simulink model "MultiIntersectionStoplight"  (R2020a)
settings: Solver=VariableStepAuto  StartTime=0.0  StopTime=inf  RelTol=1e-3
libraries: dspnetwork x119, sldrtlib x1
settings Model: Creator=brandon  LastModifiedBy=brandon

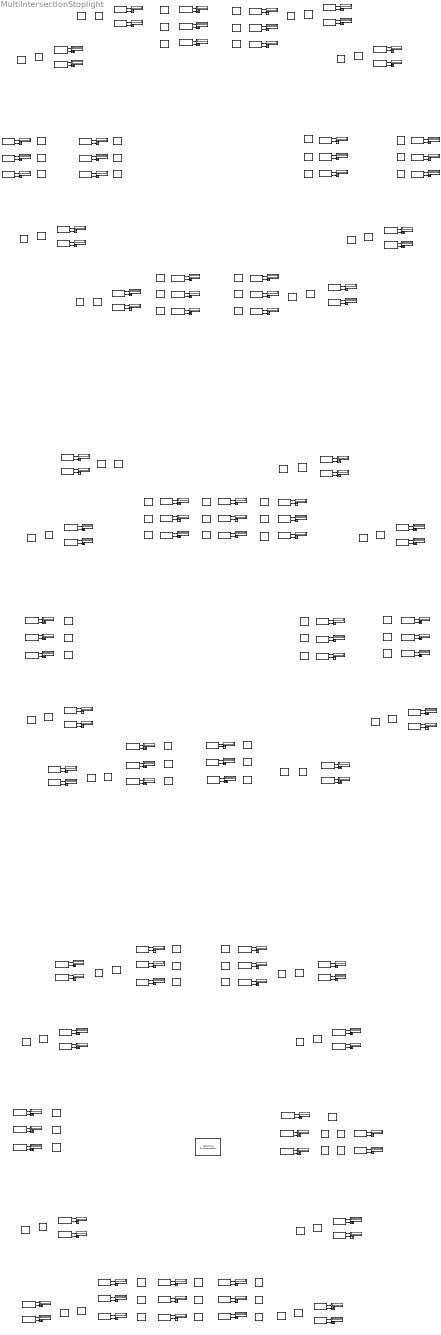
== system MultiIntersectionStoplight ==
  note: Walk: UDP 25003
      | Don't Walk: UDP 25004
  note: Walk: UDP 25005
      | Don't Walk: UDP 25006
  note: Walk: UDP 25011
      | Don't Walk: UDP 25012
  note: Walk: UDP 25013
      | Don't Walk: UDP 25014
  note: Red: UDP 26001
      | Yellow: UDP 26002
      | Green: UDP 26003
  note: Red: UDP 26004
      | Yellow: UDP 26005
      | Green: UDP 26006
  note: Red: UDP 26007
      | Yellow: UDP 26008
      | Green: UDP 26009
  note: Red: UDP 26010
      | Yellow: UDP 26011
      | Green: UDP 26012
  note: Red: UDP 26013
      | Yellow: UDP 26014
      | Green: UDP 26015
  note: Red: UDP 26016
      | Yellow: UDP 26017
      | Green: UDP 26018
  note: Red: UDP 26019
      | Yellow: UDP 26020
      | Green: UDP 26021
      | Yellow Left: UDP 26022
      | Green Left: UDP 26023
  note: Intersection of Ruggles and Huntington
      | Crosswalks: UDP Ports 25001-25016
      | Stoplights: UPD Ports 26001-26023
  note: Intersection of Parker and Huntington
      | Crosswalks: UDP Ports 25017-25032
      | Stoplights: UPD Ports 26024-26047
  note: Walk: UDP 25019
      | Don't Walk: UDP 25020
  note: Walk: UDP 25021
      | Don't Walk: UDP 25022
  note: Walk: UDP 25029
      | Don't Walk: UDP 25030
  note: Walk: UDP 25027
      | Don't Walk: UDP 25028
  note: Red: UDP 26024
      | Yellow: UDP 26025
      | Green: UDP 26026
  note: Red: UDP 26027
      | Yellow: UDP 26028
      | Green: UDP 26029
  note: Red: UDP 26030
      | Yellow: UDP 26031
      | Green: UDP 26032
  note: Red: UDP 26033
      | Yellow: UDP 26034
      | Green: UDP 26035
  note: Red: UDP 26036
      | Yellow: UDP 26037
      | Green: UDP 26038
  note: Red: UDP 26039
      | Yellow: UDP 26040
      | Green: UDP 26041
  note: Red: UDP 26042
      | Yellow: UDP 26043
      | Green: UDP 26044
  note: Red: UDP 26045
      | Yellow: UDP 26046
      | Green: UDP 26047
  note: Intersection of Parker and Huntington
      | Crosswalks: UDP Ports 25033-25048
      | Stoplights: UPD Ports 26048-26071
  note: Walk: UDP 25035
      | Don't Walk: UDP 25036
  note: Walk: UDP 25037
      | Don't Walk: UDP 25038
  note: Walk: UDP 25045
      | Don't Walk: UDP 25046
  note: Walk: UDP 25043
      | Don't Walk: UDP 25044
  note: Red: UDP 26066
      | Yellow: UDP 26067
      | Green: UDP 26068
  note: Red: UDP 26069
      | Yellow: UDP 26070
      | Green: UDP 26071
  note: Red: UDP 26048
      | Yellow: UDP 26049
      | Green: UDP 26050
  note: Red: UDP 26051
      | Yellow: UDP 26052
      | Green: UDP 26053
  note: Red: UDP 26057
      | Yellow: UDP 26058
      | Green: UDP 26059
  note: Red: UDP 26054
      | Yellow: UDP 26055
      | Green: UDP 26056
  note: Red: UDP 26060
      | Yellow: UDP 26061
      | Green: UDP 26062
  note: Red: UDP 26063
      | Yellow: UDP 26064
      | Green: UDP 26065
  note: Walk: UDP 25001
      | Don't Walk: UDP 25002
  note: Walk: UDP 25015
      | Don't Walk: UDP 25016
  note: Walk: UDP 25009
      | Don't Walk: UDP 25010
  note: Walk: UDP 25007
      | Don't Walk: UDP 25008
  note: Walk: UDP 25025
      | Don't Walk: UDP 25026
  note: Walk: UDP 25031
      | Don't Walk: UDP 25032
  note: Walk: UDP 25017
      | Don't Walk: UDP 25018
  note: Walk: UDP 25023
      | Don't Walk: UDP 25024
  note: Walk: UDP 25047
      | Don't Walk: UDP 25048
  note: Walk: UDP 25033
      | Don't Walk: UDP 25034
  note: Walk: UDP 25039
      | Don't Walk: UDP 25040
  note: Walk: UDP 25041
      | Don't Walk: UDP 25042
  Display{1..119} (119 alike) : Display
  Lamp{1..119} (119 alike) : LampBlock  LabelPosition=Hide
  Real-Time Synchronization : sldrtlib/Real-Time Synchronization  SampleTime=0.1  MaxMissedTicks=1000000  ShowMissedTicks=off  YieldWhenWaiting=off
  Terminator{1..119} (119 alike) : Terminator
  UDP Receive1 : dspnetwork/UDP Receive  localURL='0.0.0.0'  localPort=26010  remoteURL='0.0.0.0'  remotePort=-1  recvBufferSize=2  dims=1  signalDatatype=uint16  isComplex=off  isVarSize=off  showBlockingTime=off  blockingTime=0  sampletime=0.1  blockPlatform=[]
  UDP Receive10 : dspnetwork/UDP Receive  localURL='0.0.0.0'  localPort=26016  remoteURL='0.0.0.0'  remotePort=-1  recvBufferSize=2  dims=1  signalDatatype=uint16  isComplex=off  isVarSize=off  showBlockingTime=off  blockingTime=0  sampletime=0.1  blockPlatform=[]
  UDP Receive100 : dspnetwork/UDP Receive  localURL='0.0.0.0'  localPort=25009  remoteURL='0.0.0.0'  remotePort=-1  recvBufferSize=2  dims=1  signalDatatype=uint16  isComplex=off  isVarSize=off  showBlockingTime=off  blockingTime=0  sampletime=0.1  blockPlatform=[]
  UDP Receive101 : dspnetwork/UDP Receive  localURL='0.0.0.0'  localPort=25010  remoteURL='0.0.0.0'  remotePort=-1  recvBufferSize=2  dims=1  signalDatatype=uint16  isComplex=off  isVarSize=off  showBlockingTime=off  blockingTime=0  sampletime=0.1  blockPlatform=[]
  UDP Receive102 : dspnetwork/UDP Receive  localURL='0.0.0.0'  localPort=25007  remoteURL='0.0.0.0'  remotePort=-1  recvBufferSize=2  dims=1  signalDatatype=uint16  isComplex=off  isVarSize=off  showBlockingTime=off  blockingTime=0  sampletime=0.1  blockPlatform=[]
  UDP Receive103 : dspnetwork/UDP Receive  localURL='0.0.0.0'  localPort=25008  remoteURL='0.0.0.0'  remotePort=-1  recvBufferSize=2  dims=1  signalDatatype=uint16  isComplex=off  isVarSize=off  showBlockingTime=off  blockingTime=0  sampletime=0.1  blockPlatform=[]
  UDP Receive104 : dspnetwork/UDP Receive  localURL='0.0.0.0'  localPort=25025  remoteURL='0.0.0.0'  remotePort=-1  recvBufferSize=2  dims=1  signalDatatype=uint16  isComplex=off  isVarSize=off  showBlockingTime=off  blockingTime=0  sampletime=0.1  blockPlatform=[]
  UDP Receive105 : dspnetwork/UDP Receive  localURL='0.0.0.0'  localPort=25026  remoteURL='0.0.0.0'  remotePort=-1  recvBufferSize=2  dims=1  signalDatatype=uint16  isComplex=off  isVarSize=off  showBlockingTime=off  blockingTime=0  sampletime=0.1  blockPlatform=[]
  UDP Receive106 : dspnetwork/UDP Receive  localURL='0.0.0.0'  localPort=25031  remoteURL='0.0.0.0'  remotePort=-1  recvBufferSize=2  dims=1  signalDatatype=uint16  isComplex=off  isVarSize=off  showBlockingTime=off  blockingTime=0  sampletime=0.1  blockPlatform=[]
  UDP Receive107 : dspnetwork/UDP Receive  localURL='0.0.0.0'  localPort=25032  remoteURL='0.0.0.0'  remotePort=-1  recvBufferSize=2  dims=1  signalDatatype=uint16  isComplex=off  isVarSize=off  showBlockingTime=off  blockingTime=0  sampletime=0.1  blockPlatform=[]
  UDP Receive108 : dspnetwork/UDP Receive  localURL='0.0.0.0'  localPort=25017  remoteURL='0.0.0.0'  remotePort=-1  recvBufferSize=2  dims=1  signalDatatype=uint16  isComplex=off  isVarSize=off  showBlockingTime=off  blockingTime=0  sampletime=0.1  blockPlatform=[]
  UDP Receive109 : dspnetwork/UDP Receive  localURL='0.0.0.0'  localPort=25018  remoteURL='0.0.0.0'  remotePort=-1  recvBufferSize=2  dims=1  signalDatatype=uint16  isComplex=off  isVarSize=off  showBlockingTime=off  blockingTime=0  sampletime=0.1  blockPlatform=[]
  UDP Receive11 : dspnetwork/UDP Receive  localURL='0.0.0.0'  localPort=26013  remoteURL='0.0.0.0'  remotePort=-1  recvBufferSize=2  dims=1  signalDatatype=uint16  isComplex=off  isVarSize=off  showBlockingTime=off  blockingTime=0  sampletime=0.1  blockPlatform=[]
  UDP Receive110 : dspnetwork/UDP Receive  localURL='0.0.0.0'  localPort=25023  remoteURL='0.0.0.0'  remotePort=-1  recvBufferSize=2  dims=1  signalDatatype=uint16  isComplex=off  isVarSize=off  showBlockingTime=off  blockingTime=0  sampletime=0.1  blockPlatform=[]
  UDP Receive111 : dspnetwork/UDP Receive  localURL='0.0.0.0'  localPort=25024  remoteURL='0.0.0.0'  remotePort=-1  recvBufferSize=2  dims=1  signalDatatype=uint16  isComplex=off  isVarSize=off  showBlockingTime=off  blockingTime=0  sampletime=0.1  blockPlatform=[]
  UDP Receive112 : dspnetwork/UDP Receive  localURL='0.0.0.0'  localPort=25047  remoteURL='0.0.0.0'  remotePort=-1  recvBufferSize=2  dims=1  signalDatatype=uint16  isComplex=off  isVarSize=off  showBlockingTime=off  blockingTime=0  sampletime=0.1  blockPlatform=[]
  UDP Receive113 : dspnetwork/UDP Receive  localURL='0.0.0.0'  localPort=25048  remoteURL='0.0.0.0'  remotePort=-1  recvBufferSize=2  dims=1  signalDatatype=uint16  isComplex=off  isVarSize=off  showBlockingTime=off  blockingTime=0  sampletime=0.1  blockPlatform=[]
  UDP Receive114 : dspnetwork/UDP Receive  localURL='0.0.0.0'  localPort=25033  remoteURL='0.0.0.0'  remotePort=-1  recvBufferSize=2  dims=1  signalDatatype=uint16  isComplex=off  isVarSize=off  showBlockingTime=off  blockingTime=0  sampletime=0.1  blockPlatform=[]
  UDP Receive115 : dspnetwork/UDP Receive  localURL='0.0.0.0'  localPort=25034  remoteURL='0.0.0.0'  remotePort=-1  recvBufferSize=2  dims=1  signalDatatype=uint16  isComplex=off  isVarSize=off  showBlockingTime=off  blockingTime=0  sampletime=0.1  blockPlatform=[]
  UDP Receive116 : dspnetwork/UDP Receive  localURL='0.0.0.0'  localPort=25039  remoteURL='0.0.0.0'  remotePort=-1  recvBufferSize=2  dims=1  signalDatatype=uint16  isComplex=off  isVarSize=off  showBlockingTime=off  blockingTime=0  sampletime=0.1  blockPlatform=[]
  UDP Receive117 : dspnetwork/UDP Receive  localURL='0.0.0.0'  localPort=25040  remoteURL='0.0.0.0'  remotePort=-1  recvBufferSize=2  dims=1  signalDatatype=uint16  isComplex=off  isVarSize=off  showBlockingTime=off  blockingTime=0  sampletime=0.1  blockPlatform=[]
  UDP Receive118 : dspnetwork/UDP Receive  localURL='0.0.0.0'  localPort=25041  remoteURL='0.0.0.0'  remotePort=-1  recvBufferSize=2  dims=1  signalDatatype=uint16  isComplex=off  isVarSize=off  showBlockingTime=off  blockingTime=0  sampletime=0.1  blockPlatform=[]
  UDP Receive119 : dspnetwork/UDP Receive  localURL='0.0.0.0'  localPort=25042  remoteURL='0.0.0.0'  remotePort=-1  recvBufferSize=2  dims=1  signalDatatype=uint16  isComplex=off  isVarSize=off  showBlockingTime=off  blockingTime=0  sampletime=0.1  blockPlatform=[]
  UDP Receive12 : dspnetwork/UDP Receive  localURL='0.0.0.0'  localPort=26007  remoteURL='0.0.0.0'  remotePort=-1  recvBufferSize=2  dims=1  signalDatatype=uint16  isComplex=off  isVarSize=off  showBlockingTime=off  blockingTime=0  sampletime=0.1  blockPlatform=[]
  UDP Receive13 : dspnetwork/UDP Receive  localURL='0.0.0.0'  localPort=26008  remoteURL='0.0.0.0'  remotePort=-1  recvBufferSize=2  dims=1  signalDatatype=uint16  isComplex=off  isVarSize=off  showBlockingTime=off  blockingTime=0  sampletime=0.1  blockPlatform=[]
  UDP Receive14 : dspnetwork/UDP Receive  localURL='0.0.0.0'  localPort=26009  remoteURL='0.0.0.0'  remotePort=-1  recvBufferSize=2  dims=1  signalDatatype=uint16  isComplex=off  isVarSize=off  showBlockingTime=off  blockingTime=0  sampletime=0.1  blockPlatform=[]
  UDP Receive15 : dspnetwork/UDP Receive  localURL='0.0.0.0'  localPort=26004  remoteURL='0.0.0.0'  remotePort=-1  recvBufferSize=2  dims=1  signalDatatype=uint16  isComplex=off  isVarSize=off  showBlockingTime=off  blockingTime=0  sampletime=0.1  blockPlatform=[]
  UDP Receive16 : dspnetwork/UDP Receive  localURL='0.0.0.0'  localPort=26005  remoteURL='0.0.0.0'  remotePort=-1  recvBufferSize=2  dims=1  signalDatatype=uint16  isComplex=off  isVarSize=off  showBlockingTime=off  blockingTime=0  sampletime=0.1  blockPlatform=[]
  UDP Receive17 : dspnetwork/UDP Receive  localURL='0.0.0.0'  localPort=26006  remoteURL='0.0.0.0'  remotePort=-1  recvBufferSize=2  dims=1  signalDatatype=uint16  isComplex=off  isVarSize=off  showBlockingTime=off  blockingTime=0  sampletime=0.1  blockPlatform=[]
  UDP Receive18 : dspnetwork/UDP Receive  localURL='0.0.0.0'  localPort=26001  remoteURL='0.0.0.0'  remotePort=-1  recvBufferSize=2  dims=1  signalDatatype=uint16  isComplex=off  isVarSize=off  showBlockingTime=off  blockingTime=0  sampletime=0.1  blockPlatform=[]
  UDP Receive19 : dspnetwork/UDP Receive  localURL='0.0.0.0'  localPort=26002  remoteURL='0.0.0.0'  remotePort=-1  recvBufferSize=2  dims=1  signalDatatype=uint16  isComplex=off  isVarSize=off  showBlockingTime=off  blockingTime=0  sampletime=0.1  blockPlatform=[]
  UDP Receive2 : dspnetwork/UDP Receive  localURL='0.0.0.0'  localPort=26011  remoteURL='0.0.0.0'  remotePort=-1  recvBufferSize=2  dims=1  signalDatatype=uint16  isComplex=off  isVarSize=off  showBlockingTime=off  blockingTime=0  sampletime=0.1  blockPlatform=[]
  UDP Receive20 : dspnetwork/UDP Receive  localURL='0.0.0.0'  localPort=26003  remoteURL='0.0.0.0'  remotePort=-1  recvBufferSize=2  dims=1  signalDatatype=uint16  isComplex=off  isVarSize=off  showBlockingTime=off  blockingTime=0  sampletime=0.1  blockPlatform=[]
  UDP Receive21 : dspnetwork/UDP Receive  localURL='0.0.0.0'  localPort=25005  remoteURL='0.0.0.0'  remotePort=-1  recvBufferSize=2  dims=1  signalDatatype=uint16  isComplex=off  isVarSize=off  showBlockingTime=off  blockingTime=0  sampletime=0.1  blockPlatform=[]
  UDP Receive22 : dspnetwork/UDP Receive  localURL='0.0.0.0'  localPort=25006  remoteURL='0.0.0.0'  remotePort=-1  recvBufferSize=2  dims=1  signalDatatype=uint16  isComplex=off  isVarSize=off  showBlockingTime=off  blockingTime=0  sampletime=0.1  blockPlatform=[]
  UDP Receive23 : dspnetwork/UDP Receive  localURL='0.0.0.0'  localPort=25003  remoteURL='0.0.0.0'  remotePort=-1  recvBufferSize=2  dims=1  signalDatatype=uint16  isComplex=off  isVarSize=off  showBlockingTime=off  blockingTime=0  sampletime=0.1  blockPlatform=[]
  UDP Receive24 : dspnetwork/UDP Receive  localURL='0.0.0.0'  localPort=25004  remoteURL='0.0.0.0'  remotePort=-1  recvBufferSize=2  dims=1  signalDatatype=uint16  isComplex=off  isVarSize=off  showBlockingTime=off  blockingTime=0  sampletime=0.1  blockPlatform=[]
  UDP Receive25 : dspnetwork/UDP Receive  localURL='0.0.0.0'  localPort=26021  remoteURL='0.0.0.0'  remotePort=-1  recvBufferSize=2  dims=1  signalDatatype=uint16  isComplex=off  isVarSize=off  showBlockingTime=off  blockingTime=0  sampletime=0.1  blockPlatform=[]
  UDP Receive26 : dspnetwork/UDP Receive  localURL='0.0.0.0'  localPort=26020  remoteURL='0.0.0.0'  remotePort=-1  recvBufferSize=2  dims=1  signalDatatype=uint16  isComplex=off  isVarSize=off  showBlockingTime=off  blockingTime=0  sampletime=0.1  blockPlatform=[]
  UDP Receive27 : dspnetwork/UDP Receive  localURL='0.0.0.0'  localPort=26023  remoteURL='0.0.0.0'  remotePort=-1  recvBufferSize=2  dims=1  signalDatatype=uint16  isComplex=off  isVarSize=off  showBlockingTime=off  blockingTime=0  sampletime=0.1  blockPlatform=[]
  UDP Receive28 : dspnetwork/UDP Receive  localURL='0.0.0.0'  localPort=26022  remoteURL='0.0.0.0'  remotePort=-1  recvBufferSize=2  dims=1  signalDatatype=uint16  isComplex=off  isVarSize=off  showBlockingTime=off  blockingTime=0  sampletime=0.1  blockPlatform=[]
  UDP Receive29 : dspnetwork/UDP Receive  localURL='0.0.0.0'  localPort=26019  remoteURL='0.0.0.0'  remotePort=-1  recvBufferSize=2  dims=1  signalDatatype=uint16  isComplex=off  isVarSize=off  showBlockingTime=off  blockingTime=0  sampletime=0.1  blockPlatform=[]
  UDP Receive3 : dspnetwork/UDP Receive  localURL='0.0.0.0'  localPort=25013  remoteURL='0.0.0.0'  remotePort=-1  recvBufferSize=2  dims=1  signalDatatype=uint16  isComplex=off  isVarSize=off  showBlockingTime=off  blockingTime=0  sampletime=0.1  blockPlatform=[]
  UDP Receive30 : dspnetwork/UDP Receive  localURL='0.0.0.0'  localPort=26014  remoteURL='0.0.0.0'  remotePort=-1  recvBufferSize=2  dims=1  signalDatatype=uint16  isComplex=off  isVarSize=off  showBlockingTime=off  blockingTime=0  sampletime=0.1  blockPlatform=[]
  UDP Receive31 : dspnetwork/UDP Receive  localURL='0.0.0.0'  localPort=26015  remoteURL='0.0.0.0'  remotePort=-1  recvBufferSize=2  dims=1  signalDatatype=uint16  isComplex=off  isVarSize=off  showBlockingTime=off  blockingTime=0  sampletime=0.1  blockPlatform=[]
  UDP Receive32 : dspnetwork/UDP Receive  localURL='0.0.0.0'  localPort=25019  remoteURL='0.0.0.0'  remotePort=-1  recvBufferSize=2  dims=1  signalDatatype=uint16  isComplex=off  isVarSize=off  showBlockingTime=off  blockingTime=0  sampletime=0.1  blockPlatform=[]
  UDP Receive33 : dspnetwork/UDP Receive  localURL='0.0.0.0'  localPort=25020  remoteURL='0.0.0.0'  remotePort=-1  recvBufferSize=2  dims=1  signalDatatype=uint16  isComplex=off  isVarSize=off  showBlockingTime=off  blockingTime=0  sampletime=0.1  blockPlatform=[]
  UDP Receive34 : dspnetwork/UDP Receive  localURL='0.0.0.0'  localPort=25021  remoteURL='0.0.0.0'  remotePort=-1  recvBufferSize=2  dims=1  signalDatatype=uint16  isComplex=off  isVarSize=off  showBlockingTime=off  blockingTime=0  sampletime=0.1  blockPlatform=[]
  UDP Receive35 : dspnetwork/UDP Receive  localURL='0.0.0.0'  localPort=25022  remoteURL='0.0.0.0'  remotePort=-1  recvBufferSize=2  dims=1  signalDatatype=uint16  isComplex=off  isVarSize=off  showBlockingTime=off  blockingTime=0  sampletime=0.1  blockPlatform=[]
  UDP Receive36 : dspnetwork/UDP Receive  localURL='0.0.0.0'  localPort=25027  remoteURL='0.0.0.0'  remotePort=-1  recvBufferSize=2  dims=1  signalDatatype=uint16  isComplex=off  isVarSize=off  showBlockingTime=off  blockingTime=0  sampletime=0.1  blockPlatform=[]
  UDP Receive37 : dspnetwork/UDP Receive  localURL='0.0.0.0'  localPort=25028  remoteURL='0.0.0.0'  remotePort=-1  recvBufferSize=2  dims=1  signalDatatype=uint16  isComplex=off  isVarSize=off  showBlockingTime=off  blockingTime=0  sampletime=0.1  blockPlatform=[]
  UDP Receive38 : dspnetwork/UDP Receive  localURL='0.0.0.0'  localPort=25029  remoteURL='0.0.0.0'  remotePort=-1  recvBufferSize=2  dims=1  signalDatatype=uint16  isComplex=off  isVarSize=off  showBlockingTime=off  blockingTime=0  sampletime=0.1  blockPlatform=[]
  UDP Receive39 : dspnetwork/UDP Receive  localURL='0.0.0.0'  localPort=25030  remoteURL='0.0.0.0'  remotePort=-1  recvBufferSize=2  dims=1  signalDatatype=uint16  isComplex=off  isVarSize=off  showBlockingTime=off  blockingTime=0  sampletime=0.1  blockPlatform=[]
  UDP Receive4 : dspnetwork/UDP Receive  localURL='0.0.0.0'  localPort=25014  remoteURL='0.0.0.0'  remotePort=-1  recvBufferSize=2  dims=1  signalDatatype=uint16  isComplex=off  isVarSize=off  showBlockingTime=off  blockingTime=0  sampletime=0.1  blockPlatform=[]
  UDP Receive40 : dspnetwork/UDP Receive  localURL='0.0.0.0'  localPort=26027  remoteURL='0.0.0.0'  remotePort=-1  recvBufferSize=2  dims=1  signalDatatype=uint16  isComplex=off  isVarSize=off  showBlockingTime=off  blockingTime=0  sampletime=0.1  blockPlatform=[]
  UDP Receive41 : dspnetwork/UDP Receive  localURL='0.0.0.0'  localPort=26028  remoteURL='0.0.0.0'  remotePort=-1  recvBufferSize=2  dims=1  signalDatatype=uint16  isComplex=off  isVarSize=off  showBlockingTime=off  blockingTime=0  sampletime=0.1  blockPlatform=[]
  UDP Receive42 : dspnetwork/UDP Receive  localURL='0.0.0.0'  localPort=26029  remoteURL='0.0.0.0'  remotePort=-1  recvBufferSize=2  dims=1  signalDatatype=uint16  isComplex=off  isVarSize=off  showBlockingTime=off  blockingTime=0  sampletime=0.1  blockPlatform=[]
  UDP Receive43 : dspnetwork/UDP Receive  localURL='0.0.0.0'  localPort=26024  remoteURL='0.0.0.0'  remotePort=-1  recvBufferSize=2  dims=1  signalDatatype=uint16  isComplex=off  isVarSize=off  showBlockingTime=off  blockingTime=0  sampletime=0.1  blockPlatform=[]
  UDP Receive44 : dspnetwork/UDP Receive  localURL='0.0.0.0'  localPort=26025  remoteURL='0.0.0.0'  remotePort=-1  recvBufferSize=2  dims=1  signalDatatype=uint16  isComplex=off  isVarSize=off  showBlockingTime=off  blockingTime=0  sampletime=0.1  blockPlatform=[]
  UDP Receive45 : dspnetwork/UDP Receive  localURL='0.0.0.0'  localPort=26026  remoteURL='0.0.0.0'  remotePort=-1  recvBufferSize=2  dims=1  signalDatatype=uint16  isComplex=off  isVarSize=off  showBlockingTime=off  blockingTime=0  sampletime=0.1  blockPlatform=[]
  UDP Receive46 : dspnetwork/UDP Receive  localURL='0.0.0.0'  localPort=26030  remoteURL='0.0.0.0'  remotePort=-1  recvBufferSize=2  dims=1  signalDatatype=uint16  isComplex=off  isVarSize=off  showBlockingTime=off  blockingTime=0  sampletime=0.1  blockPlatform=[]
  UDP Receive47 : dspnetwork/UDP Receive  localURL='0.0.0.0'  localPort=26031  remoteURL='0.0.0.0'  remotePort=-1  recvBufferSize=2  dims=1  signalDatatype=uint16  isComplex=off  isVarSize=off  showBlockingTime=off  blockingTime=0  sampletime=0.1  blockPlatform=[]
  UDP Receive48 : dspnetwork/UDP Receive  localURL='0.0.0.0'  localPort=26032  remoteURL='0.0.0.0'  remotePort=-1  recvBufferSize=2  dims=1  signalDatatype=uint16  isComplex=off  isVarSize=off  showBlockingTime=off  blockingTime=0  sampletime=0.1  blockPlatform=[]
  UDP Receive49 : dspnetwork/UDP Receive  localURL='0.0.0.0'  localPort=26044  remoteURL='0.0.0.0'  remotePort=-1  recvBufferSize=2  dims=1  signalDatatype=uint16  isComplex=off  isVarSize=off  showBlockingTime=off  blockingTime=0  sampletime=0.1  blockPlatform=[]
  UDP Receive5 : dspnetwork/UDP Receive  localURL='0.0.0.0'  localPort=26018  remoteURL='0.0.0.0'  remotePort=-1  recvBufferSize=2  dims=1  signalDatatype=uint16  isComplex=off  isVarSize=off  showBlockingTime=off  blockingTime=0  sampletime=0.1  blockPlatform=[]
  UDP Receive50 : dspnetwork/UDP Receive  localURL='0.0.0.0'  localPort=26043  remoteURL='0.0.0.0'  remotePort=-1  recvBufferSize=2  dims=1  signalDatatype=uint16  isComplex=off  isVarSize=off  showBlockingTime=off  blockingTime=0  sampletime=0.1  blockPlatform=[]
  UDP Receive51 : dspnetwork/UDP Receive  localURL='0.0.0.0'  localPort=26042  remoteURL='0.0.0.0'  remotePort=-1  recvBufferSize=2  dims=1  signalDatatype=uint16  isComplex=off  isVarSize=off  showBlockingTime=off  blockingTime=0  sampletime=0.1  blockPlatform=[]
  UDP Receive52 : dspnetwork/UDP Receive  localURL='0.0.0.0'  localPort=26047  remoteURL='0.0.0.0'  remotePort=-1  recvBufferSize=2  dims=1  signalDatatype=uint16  isComplex=off  isVarSize=off  showBlockingTime=off  blockingTime=0  sampletime=0.1  blockPlatform=[]
  UDP Receive53 : dspnetwork/UDP Receive  localURL='0.0.0.0'  localPort=26046  remoteURL='0.0.0.0'  remotePort=-1  recvBufferSize=2  dims=1  signalDatatype=uint16  isComplex=off  isVarSize=off  showBlockingTime=off  blockingTime=0  sampletime=0.1  blockPlatform=[]
  UDP Receive54 : dspnetwork/UDP Receive  localURL='0.0.0.0'  localPort=26045  remoteURL='0.0.0.0'  remotePort=-1  recvBufferSize=2  dims=1  signalDatatype=uint16  isComplex=off  isVarSize=off  showBlockingTime=off  blockingTime=0  sampletime=0.1  blockPlatform=[]
  UDP Receive55 : dspnetwork/UDP Receive  localURL='0.0.0.0'  localPort=26039  remoteURL='0.0.0.0'  remotePort=-1  recvBufferSize=2  dims=1  signalDatatype=uint16  isComplex=off  isVarSize=off  showBlockingTime=off  blockingTime=0  sampletime=0.1  blockPlatform=[]
  UDP Receive56 : dspnetwork/UDP Receive  localURL='0.0.0.0'  localPort=26040  remoteURL='0.0.0.0'  remotePort=-1  recvBufferSize=2  dims=1  signalDatatype=uint16  isComplex=off  isVarSize=off  showBlockingTime=off  blockingTime=0  sampletime=0.1  blockPlatform=[]
  UDP Receive57 : dspnetwork/UDP Receive  localURL='0.0.0.0'  localPort=26041  remoteURL='0.0.0.0'  remotePort=-1  recvBufferSize=2  dims=1  signalDatatype=uint16  isComplex=off  isVarSize=off  showBlockingTime=off  blockingTime=0  sampletime=0.1  blockPlatform=[]
  UDP Receive58 : dspnetwork/UDP Receive  localURL='0.0.0.0'  localPort=26036  remoteURL='0.0.0.0'  remotePort=-1  recvBufferSize=2  dims=1  signalDatatype=uint16  isComplex=off  isVarSize=off  showBlockingTime=off  blockingTime=0  sampletime=0.1  blockPlatform=[]
  UDP Receive59 : dspnetwork/UDP Receive  localURL='0.0.0.0'  localPort=26037  remoteURL='0.0.0.0'  remotePort=-1  recvBufferSize=2  dims=1  signalDatatype=uint16  isComplex=off  isVarSize=off  showBlockingTime=off  blockingTime=0  sampletime=0.1  blockPlatform=[]
  UDP Receive6 : dspnetwork/UDP Receive  localURL='0.0.0.0'  localPort=26012  remoteURL='0.0.0.0'  remotePort=-1  recvBufferSize=2  dims=1  signalDatatype=uint16  isComplex=off  isVarSize=off  showBlockingTime=off  blockingTime=0  sampletime=0.1  blockPlatform=[]
  UDP Receive60 : dspnetwork/UDP Receive  localURL='0.0.0.0'  localPort=26038  remoteURL='0.0.0.0'  remotePort=-1  recvBufferSize=2  dims=1  signalDatatype=uint16  isComplex=off  isVarSize=off  showBlockingTime=off  blockingTime=0  sampletime=0.1  blockPlatform=[]
  UDP Receive61 : dspnetwork/UDP Receive  localURL='0.0.0.0'  localPort=26033  remoteURL='0.0.0.0'  remotePort=-1  recvBufferSize=2  dims=1  signalDatatype=uint16  isComplex=off  isVarSize=off  showBlockingTime=off  blockingTime=0  sampletime=0.1  blockPlatform=[]
  UDP Receive62 : dspnetwork/UDP Receive  localURL='0.0.0.0'  localPort=26034  remoteURL='0.0.0.0'  remotePort=-1  recvBufferSize=2  dims=1  signalDatatype=uint16  isComplex=off  isVarSize=off  showBlockingTime=off  blockingTime=0  sampletime=0.1  blockPlatform=[]
  UDP Receive63 : dspnetwork/UDP Receive  localURL='0.0.0.0'  localPort=26035  remoteURL='0.0.0.0'  remotePort=-1  recvBufferSize=2  dims=1  signalDatatype=uint16  isComplex=off  isVarSize=off  showBlockingTime=off  blockingTime=0  sampletime=0.1  blockPlatform=[]
  UDP Receive64 : dspnetwork/UDP Receive  localURL='0.0.0.0'  localPort=26062  remoteURL='0.0.0.0'  remotePort=-1  recvBufferSize=2  dims=1  signalDatatype=uint16  isComplex=off  isVarSize=off  showBlockingTime=off  blockingTime=0  sampletime=0.1  blockPlatform=[]
  UDP Receive65 : dspnetwork/UDP Receive  localURL='0.0.0.0'  localPort=26061  remoteURL='0.0.0.0'  remotePort=-1  recvBufferSize=2  dims=1  signalDatatype=uint16  isComplex=off  isVarSize=off  showBlockingTime=off  blockingTime=0  sampletime=0.1  blockPlatform=[]
  UDP Receive66 : dspnetwork/UDP Receive  localURL='0.0.0.0'  localPort=26060  remoteURL='0.0.0.0'  remotePort=-1  recvBufferSize=2  dims=1  signalDatatype=uint16  isComplex=off  isVarSize=off  showBlockingTime=off  blockingTime=0  sampletime=0.1  blockPlatform=[]
  UDP Receive67 : dspnetwork/UDP Receive  localURL='0.0.0.0'  localPort=26065  remoteURL='0.0.0.0'  remotePort=-1  recvBufferSize=2  dims=1  signalDatatype=uint16  isComplex=off  isVarSize=off  showBlockingTime=off  blockingTime=0  sampletime=0.1  blockPlatform=[]
  UDP Receive68 : dspnetwork/UDP Receive  localURL='0.0.0.0'  localPort=26064  remoteURL='0.0.0.0'  remotePort=-1  recvBufferSize=2  dims=1  signalDatatype=uint16  isComplex=off  isVarSize=off  showBlockingTime=off  blockingTime=0  sampletime=0.1  blockPlatform=[]
  UDP Receive69 : dspnetwork/UDP Receive  localURL='0.0.0.0'  localPort=26063  remoteURL='0.0.0.0'  remotePort=-1  recvBufferSize=2  dims=1  signalDatatype=uint16  isComplex=off  isVarSize=off  showBlockingTime=off  blockingTime=0  sampletime=0.1  blockPlatform=[]
  UDP Receive7 : dspnetwork/UDP Receive  localURL='0.0.0.0'  localPort=25012  remoteURL='0.0.0.0'  remotePort=-1  recvBufferSize=2  dims=1  signalDatatype=uint16  isComplex=off  isVarSize=off  showBlockingTime=off  blockingTime=0  sampletime=0.1  blockPlatform=[]
  UDP Receive70 : dspnetwork/UDP Receive  localURL='0.0.0.0'  localPort=26056  remoteURL='0.0.0.0'  remotePort=-1  recvBufferSize=2  dims=1  signalDatatype=uint16  isComplex=off  isVarSize=off  showBlockingTime=off  blockingTime=0  sampletime=0.1  blockPlatform=[]
  UDP Receive71 : dspnetwork/UDP Receive  localURL='0.0.0.0'  localPort=26055  remoteURL='0.0.0.0'  remotePort=-1  recvBufferSize=2  dims=1  signalDatatype=uint16  isComplex=off  isVarSize=off  showBlockingTime=off  blockingTime=0  sampletime=0.1  blockPlatform=[]
  UDP Receive72 : dspnetwork/UDP Receive  localURL='0.0.0.0'  localPort=26054  remoteURL='0.0.0.0'  remotePort=-1  recvBufferSize=2  dims=1  signalDatatype=uint16  isComplex=off  isVarSize=off  showBlockingTime=off  blockingTime=0  sampletime=0.1  blockPlatform=[]
  UDP Receive73 : dspnetwork/UDP Receive  localURL='0.0.0.0'  localPort=26059  remoteURL='0.0.0.0'  remotePort=-1  recvBufferSize=2  dims=1  signalDatatype=uint16  isComplex=off  isVarSize=off  showBlockingTime=off  blockingTime=0  sampletime=0.1  blockPlatform=[]
  UDP Receive74 : dspnetwork/UDP Receive  localURL='0.0.0.0'  localPort=26058  remoteURL='0.0.0.0'  remotePort=-1  recvBufferSize=2  dims=1  signalDatatype=uint16  isComplex=off  isVarSize=off  showBlockingTime=off  blockingTime=0  sampletime=0.1  blockPlatform=[]
  UDP Receive75 : dspnetwork/UDP Receive  localURL='0.0.0.0'  localPort=26057  remoteURL='0.0.0.0'  remotePort=-1  recvBufferSize=2  dims=1  signalDatatype=uint16  isComplex=off  isVarSize=off  showBlockingTime=off  blockingTime=0  sampletime=0.1  blockPlatform=[]
  UDP Receive76 : dspnetwork/UDP Receive  localURL='0.0.0.0'  localPort=26068  remoteURL='0.0.0.0'  remotePort=-1  recvBufferSize=2  dims=1  signalDatatype=uint16  isComplex=off  isVarSize=off  showBlockingTime=off  blockingTime=0  sampletime=0.1  blockPlatform=[]
  UDP Receive77 : dspnetwork/UDP Receive  localURL='0.0.0.0'  localPort=26067  remoteURL='0.0.0.0'  remotePort=-1  recvBufferSize=2  dims=1  signalDatatype=uint16  isComplex=off  isVarSize=off  showBlockingTime=off  blockingTime=0  sampletime=0.1  blockPlatform=[]
  UDP Receive78 : dspnetwork/UDP Receive  localURL='0.0.0.0'  localPort=26066  remoteURL='0.0.0.0'  remotePort=-1  recvBufferSize=2  dims=1  signalDatatype=uint16  isComplex=off  isVarSize=off  showBlockingTime=off  blockingTime=0  sampletime=0.1  blockPlatform=[]
  UDP Receive79 : dspnetwork/UDP Receive  localURL='0.0.0.0'  localPort=26071  remoteURL='0.0.0.0'  remotePort=-1  recvBufferSize=2  dims=1  signalDatatype=uint16  isComplex=off  isVarSize=off  showBlockingTime=off  blockingTime=0  sampletime=0.1  blockPlatform=[]
  UDP Receive8 : dspnetwork/UDP Receive  localURL='0.0.0.0'  localPort=25011  remoteURL='0.0.0.0'  remotePort=-1  recvBufferSize=2  dims=1  signalDatatype=uint16  isComplex=off  isVarSize=off  showBlockingTime=off  blockingTime=0  sampletime=0.1  blockPlatform=[]
  UDP Receive80 : dspnetwork/UDP Receive  localURL='0.0.0.0'  localPort=26070  remoteURL='0.0.0.0'  remotePort=-1  recvBufferSize=2  dims=1  signalDatatype=uint16  isComplex=off  isVarSize=off  showBlockingTime=off  blockingTime=0  sampletime=0.1  blockPlatform=[]
  UDP Receive81 : dspnetwork/UDP Receive  localURL='0.0.0.0'  localPort=26069  remoteURL='0.0.0.0'  remotePort=-1  recvBufferSize=2  dims=1  signalDatatype=uint16  isComplex=off  isVarSize=off  showBlockingTime=off  blockingTime=0  sampletime=0.1  blockPlatform=[]
  UDP Receive82 : dspnetwork/UDP Receive  localURL='0.0.0.0'  localPort=26053  remoteURL='0.0.0.0'  remotePort=-1  recvBufferSize=2  dims=1  signalDatatype=uint16  isComplex=off  isVarSize=off  showBlockingTime=off  blockingTime=0  sampletime=0.1  blockPlatform=[]
  UDP Receive83 : dspnetwork/UDP Receive  localURL='0.0.0.0'  localPort=26052  remoteURL='0.0.0.0'  remotePort=-1  recvBufferSize=2  dims=1  signalDatatype=uint16  isComplex=off  isVarSize=off  showBlockingTime=off  blockingTime=0  sampletime=0.1  blockPlatform=[]
  UDP Receive84 : dspnetwork/UDP Receive  localURL='0.0.0.0'  localPort=26051  remoteURL='0.0.0.0'  remotePort=-1  recvBufferSize=2  dims=1  signalDatatype=uint16  isComplex=off  isVarSize=off  showBlockingTime=off  blockingTime=0  sampletime=0.1  blockPlatform=[]
  UDP Receive85 : dspnetwork/UDP Receive  localURL='0.0.0.0'  localPort=26050  remoteURL='0.0.0.0'  remotePort=-1  recvBufferSize=2  dims=1  signalDatatype=uint16  isComplex=off  isVarSize=off  showBlockingTime=off  blockingTime=0  sampletime=0.1  blockPlatform=[]
  UDP Receive86 : dspnetwork/UDP Receive  localURL='0.0.0.0'  localPort=26049  remoteURL='0.0.0.0'  remotePort=-1  recvBufferSize=2  dims=1  signalDatatype=uint16  isComplex=off  isVarSize=off  showBlockingTime=off  blockingTime=0  sampletime=0.1  blockPlatform=[]
  UDP Receive87 : dspnetwork/UDP Receive  localURL='0.0.0.0'  localPort=26048  remoteURL='0.0.0.0'  remotePort=-1  recvBufferSize=2  dims=1  signalDatatype=uint16  isComplex=off  isVarSize=off  showBlockingTime=off  blockingTime=0  sampletime=0.1  blockPlatform=[]
  UDP Receive88 : dspnetwork/UDP Receive  localURL='0.0.0.0'  localPort=25035  remoteURL='0.0.0.0'  remotePort=-1  recvBufferSize=2  dims=1  signalDatatype=uint16  isComplex=off  isVarSize=off  showBlockingTime=off  blockingTime=0  sampletime=0.1  blockPlatform=[]
  UDP Receive89 : dspnetwork/UDP Receive  localURL='0.0.0.0'  localPort=25036  remoteURL='0.0.0.0'  remotePort=-1  recvBufferSize=2  dims=1  signalDatatype=uint16  isComplex=off  isVarSize=off  showBlockingTime=off  blockingTime=0  sampletime=0.1  blockPlatform=[]
  UDP Receive9 : dspnetwork/UDP Receive  localURL='0.0.0.0'  localPort=26017  remoteURL='0.0.0.0'  remotePort=-1  recvBufferSize=2  dims=1  signalDatatype=uint16  isComplex=off  isVarSize=off  showBlockingTime=off  blockingTime=0  sampletime=0.1  blockPlatform=[]
  UDP Receive90 : dspnetwork/UDP Receive  localURL='0.0.0.0'  localPort=25037  remoteURL='0.0.0.0'  remotePort=-1  recvBufferSize=2  dims=1  signalDatatype=uint16  isComplex=off  isVarSize=off  showBlockingTime=off  blockingTime=0  sampletime=0.1  blockPlatform=[]
  UDP Receive91 : dspnetwork/UDP Receive  localURL='0.0.0.0'  localPort=25038  remoteURL='0.0.0.0'  remotePort=-1  recvBufferSize=2  dims=1  signalDatatype=uint16  isComplex=off  isVarSize=off  showBlockingTime=off  blockingTime=0  sampletime=0.1  blockPlatform=[]
  UDP Receive92 : dspnetwork/UDP Receive  localURL='0.0.0.0'  localPort=25043  remoteURL='0.0.0.0'  remotePort=-1  recvBufferSize=2  dims=1  signalDatatype=uint16  isComplex=off  isVarSize=off  showBlockingTime=off  blockingTime=0  sampletime=0.1  blockPlatform=[]
  UDP Receive93 : dspnetwork/UDP Receive  localURL='0.0.0.0'  localPort=25044  remoteURL='0.0.0.0'  remotePort=-1  recvBufferSize=2  dims=1  signalDatatype=uint16  isComplex=off  isVarSize=off  showBlockingTime=off  blockingTime=0  sampletime=0.1  blockPlatform=[]
  UDP Receive94 : dspnetwork/UDP Receive  localURL='0.0.0.0'  localPort=25045  remoteURL='0.0.0.0'  remotePort=-1  recvBufferSize=2  dims=1  signalDatatype=uint16  isComplex=off  isVarSize=off  showBlockingTime=off  blockingTime=0  sampletime=0.1  blockPlatform=[]
  UDP Receive95 : dspnetwork/UDP Receive  localURL='0.0.0.0'  localPort=25046  remoteURL='0.0.0.0'  remotePort=-1  recvBufferSize=2  dims=1  signalDatatype=uint16  isComplex=off  isVarSize=off  showBlockingTime=off  blockingTime=0  sampletime=0.1  blockPlatform=[]
  UDP Receive96 : dspnetwork/UDP Receive  localURL='0.0.0.0'  localPort=25001  remoteURL='0.0.0.0'  remotePort=-1  recvBufferSize=2  dims=1  signalDatatype=uint16  isComplex=off  isVarSize=off  showBlockingTime=off  blockingTime=0  sampletime=0.1  blockPlatform=[]
  UDP Receive97 : dspnetwork/UDP Receive  localURL='0.0.0.0'  localPort=25002  remoteURL='0.0.0.0'  remotePort=-1  recvBufferSize=2  dims=1  signalDatatype=uint16  isComplex=off  isVarSize=off  showBlockingTime=off  blockingTime=0  sampletime=0.1  blockPlatform=[]
  UDP Receive98 : dspnetwork/UDP Receive  localURL='0.0.0.0'  localPort=25015  remoteURL='0.0.0.0'  remotePort=-1  recvBufferSize=2  dims=1  signalDatatype=uint16  isComplex=off  isVarSize=off  showBlockingTime=off  blockingTime=0  sampletime=0.1  blockPlatform=[]
  UDP Receive99 : dspnetwork/UDP Receive  localURL='0.0.0.0'  localPort=25016  remoteURL='0.0.0.0'  remotePort=-1  recvBufferSize=2  dims=1  signalDatatype=uint16  isComplex=off  isVarSize=off  showBlockingTime=off  blockingTime=0  sampletime=0.1  blockPlatform=[]
  wires:
  UDP Receive12/1 -> Display12/1
  UDP Receive12/2 -> Terminator12/1
  UDP Receive13/2 -> Terminator13/1
  UDP Receive13/1 -> Display13/1
  UDP Receive14/2 -> Terminator14/1
  UDP Receive14/1 -> Display14/1
  UDP Receive15/2 -> Terminator15/1
  UDP Receive15/1 -> Display15/1
  UDP Receive16/2 -> Terminator16/1
  UDP Receive16/1 -> Display16/1
  UDP Receive17/2 -> Terminator17/1
  UDP Receive17/1 -> Display17/1
  UDP Receive18/2 -> Terminator18/1
  UDP Receive18/1 -> Display18/1
  UDP Receive19/2 -> Terminator19/1
  UDP Receive19/1 -> Display19/1
  UDP Receive20/2 -> Terminator20/1
  UDP Receive20/1 -> Display20/1
  UDP Receive21/2 -> Terminator21/1
  UDP Receive21/1 -> Display21/1
  UDP Receive22/2 -> Terminator22/1
  UDP Receive22/1 -> Display22/1
  UDP Receive23/2 -> Terminator23/1
  UDP Receive23/1 -> Display23/1
  UDP Receive24/2 -> Terminator24/1
  UDP Receive24/1 -> Display24/1
  UDP Receive25/2 -> Terminator25/1
  UDP Receive25/1 -> Display25/1
  UDP Receive26/2 -> Terminator26/1
  UDP Receive26/1 -> Display26/1
  UDP Receive27/2 -> Terminator27/1
  UDP Receive27/1 -> Display27/1
  UDP Receive28/2 -> Terminator28/1
  UDP Receive28/1 -> Display28/1
  UDP Receive29/2 -> Terminator29/1
  UDP Receive29/1 -> Display29/1
  UDP Receive1/2 -> Terminator1/1
  UDP Receive1/1 -> Display1/1
  UDP Receive2/2 -> Terminator2/1
  UDP Receive2/1 -> Display2/1
  UDP Receive6/2 -> Terminator6/1
  UDP Receive6/1 -> Display6/1
  UDP Receive7/2 -> Terminator7/1
  UDP Receive7/1 -> Display7/1
  UDP Receive8/2 -> Terminator8/1
  UDP Receive8/1 -> Display8/1
  UDP Receive3/2 -> Terminator3/1
  UDP Receive3/1 -> Display3/1
  UDP Receive4/2 -> Terminator4/1
  UDP Receive4/1 -> Display4/1
  UDP Receive5/2 -> Terminator5/1
  UDP Receive5/1 -> Display5/1
  UDP Receive9/2 -> Terminator9/1
  UDP Receive9/1 -> Display9/1
  UDP Receive10/2 -> Terminator10/1
  UDP Receive10/1 -> Display10/1
  UDP Receive11/2 -> Terminator11/1
  UDP Receive11/1 -> Display11/1
  UDP Receive30/2 -> Terminator30/1
  UDP Receive30/1 -> Display30/1
  UDP Receive31/2 -> Terminator31/1
  UDP Receive31/1 -> Display31/1
  UDP Receive32/2 -> Terminator32/1
  UDP Receive32/1 -> Display32/1
  UDP Receive33/2 -> Terminator33/1
  UDP Receive33/1 -> Display33/1
  UDP Receive34/2 -> Terminator34/1
  UDP Receive34/1 -> Display34/1
  UDP Receive35/2 -> Terminator35/1
  UDP Receive35/1 -> Display35/1
  UDP Receive36/2 -> Terminator36/1
  UDP Receive36/1 -> Display36/1
  UDP Receive37/2 -> Terminator37/1
  UDP Receive37/1 -> Display37/1
  UDP Receive38/2 -> Terminator38/1
  UDP Receive38/1 -> Display38/1
  UDP Receive39/2 -> Terminator39/1
  UDP Receive39/1 -> Display39/1
  UDP Receive40/2 -> Terminator40/1
  UDP Receive40/1 -> Display40/1
  UDP Receive41/2 -> Terminator41/1
  UDP Receive41/1 -> Display41/1
  UDP Receive42/2 -> Terminator42/1
  UDP Receive42/1 -> Display42/1
  UDP Receive43/2 -> Terminator43/1
  UDP Receive43/1 -> Display43/1
  UDP Receive44/2 -> Terminator44/1
  UDP Receive44/1 -> Display44/1
  UDP Receive45/2 -> Terminator45/1
  UDP Receive45/1 -> Display45/1
  UDP Receive46/2 -> Terminator46/1
  UDP Receive46/1 -> Display46/1
  UDP Receive47/2 -> Terminator47/1
  UDP Receive47/1 -> Display47/1
  UDP Receive48/2 -> Terminator48/1
  UDP Receive48/1 -> Display48/1
  UDP Receive49/2 -> Terminator49/1
  UDP Receive49/1 -> Display49/1
  UDP Receive50/2 -> Terminator50/1
  UDP Receive50/1 -> Display50/1
  UDP Receive51/2 -> Terminator51/1
  UDP Receive51/1 -> Display51/1
  UDP Receive52/2 -> Terminator52/1
  UDP Receive52/1 -> Display52/1
  UDP Receive53/2 -> Terminator53/1
  UDP Receive53/1 -> Display53/1
  UDP Receive54/2 -> Terminator54/1
  UDP Receive54/1 -> Display54/1
  UDP Receive55/2 -> Terminator55/1
  UDP Receive55/1 -> Display55/1
  UDP Receive56/2 -> Terminator56/1
  UDP Receive56/1 -> Display56/1
  UDP Receive57/2 -> Terminator57/1
  UDP Receive57/1 -> Display57/1
  UDP Receive58/2 -> Terminator58/1
  UDP Receive58/1 -> Display58/1
  UDP Receive59/2 -> Terminator59/1
  UDP Receive59/1 -> Display59/1
  UDP Receive60/2 -> Terminator60/1
  UDP Receive60/1 -> Display60/1
  UDP Receive61/2 -> Terminator61/1
  UDP Receive61/1 -> Display61/1
  UDP Receive62/2 -> Terminator62/1
  UDP Receive62/1 -> Display62/1
  UDP Receive63/2 -> Terminator63/1
  UDP Receive63/1 -> Display63/1
  UDP Receive64/1 -> Display64/1
  UDP Receive65/1 -> Display65/1
  UDP Receive66/2 -> Terminator66/1
  UDP Receive65/2 -> Terminator65/1
  UDP Receive64/2 -> Terminator64/1
  UDP Receive66/1 -> Display66/1
  UDP Receive67/1 -> Display67/1
  UDP Receive68/1 -> Display68/1
  UDP Receive69/2 -> Terminator69/1
  UDP Receive68/2 -> Terminator68/1
  UDP Receive67/2 -> Terminator67/1
  UDP Receive69/1 -> Display69/1
  UDP Receive70/1 -> Display70/1
  UDP Receive71/1 -> Display71/1
  UDP Receive72/2 -> Terminator72/1
  UDP Receive71/2 -> Terminator71/1
  UDP Receive70/2 -> Terminator70/1
  UDP Receive72/1 -> Display72/1
  UDP Receive73/1 -> Display73/1
  UDP Receive74/1 -> Display74/1
  UDP Receive75/2 -> Terminator75/1
  UDP Receive74/2 -> Terminator74/1
  UDP Receive73/2 -> Terminator73/1
  UDP Receive75/1 -> Display75/1
  UDP Receive76/1 -> Display76/1
  UDP Receive77/1 -> Display77/1
  UDP Receive78/2 -> Terminator78/1
  UDP Receive77/2 -> Terminator77/1
  UDP Receive76/2 -> Terminator76/1
  UDP Receive78/1 -> Display78/1
  UDP Receive79/1 -> Display79/1
  UDP Receive80/1 -> Display80/1
  UDP Receive81/2 -> Terminator81/1
  UDP Receive80/2 -> Terminator80/1
  UDP Receive79/2 -> Terminator79/1
  UDP Receive81/1 -> Display81/1
  UDP Receive82/1 -> Display82/1
  UDP Receive83/1 -> Display83/1
  UDP Receive84/2 -> Terminator84/1
  UDP Receive83/2 -> Terminator83/1
  UDP Receive82/2 -> Terminator82/1
  UDP Receive84/1 -> Display84/1
  UDP Receive85/1 -> Display85/1
  UDP Receive86/1 -> Display86/1
  UDP Receive87/2 -> Terminator87/1
  UDP Receive86/2 -> Terminator86/1
  UDP Receive85/2 -> Terminator85/1
  UDP Receive87/1 -> Display87/1
  UDP Receive89/2 -> Terminator89/1
  UDP Receive89/1 -> Display89/1
  UDP Receive88/2 -> Terminator88/1
  UDP Receive88/1 -> Display88/1
  UDP Receive91/2 -> Terminator91/1
  UDP Receive91/1 -> Display91/1
  UDP Receive90/2 -> Terminator90/1
  UDP Receive90/1 -> Display90/1
  UDP Receive93/2 -> Terminator93/1
  UDP Receive93/1 -> Display93/1
  UDP Receive92/2 -> Terminator92/1
  UDP Receive92/1 -> Display92/1
  UDP Receive95/2 -> Terminator95/1
  UDP Receive95/1 -> Display95/1
  UDP Receive94/2 -> Terminator94/1
  UDP Receive94/1 -> Display94/1
  UDP Receive97/2 -> Terminator97/1
  UDP Receive96/2 -> Terminator96/1
  UDP Receive96/1 -> Display96/1
  UDP Receive97/1 -> Display97/1
  UDP Receive99/2 -> Terminator99/1
  UDP Receive98/2 -> Terminator98/1
  UDP Receive98/1 -> Display98/1
  UDP Receive99/1 -> Display99/1
  UDP Receive101/2 -> Terminator101/1
  UDP Receive100/2 -> Terminator100/1
  UDP Receive100/1 -> Display100/1
  UDP Receive101/1 -> Display101/1
  UDP Receive103/2 -> Terminator103/1
  UDP Receive102/2 -> Terminator102/1
  UDP Receive102/1 -> Display102/1
  UDP Receive103/1 -> Display103/1
  UDP Receive105/1 -> Display105/1
  UDP Receive104/2 -> Terminator104/1
  UDP Receive104/1 -> Display104/1
  UDP Receive105/2 -> Terminator105/1
  UDP Receive107/1 -> Display107/1
  UDP Receive106/2 -> Terminator106/1
  UDP Receive106/1 -> Display106/1
  UDP Receive107/2 -> Terminator107/1
  UDP Receive109/1 -> Display109/1
  UDP Receive108/2 -> Terminator108/1
  UDP Receive108/1 -> Display108/1
  UDP Receive109/2 -> Terminator109/1
  UDP Receive111/1 -> Display111/1
  UDP Receive110/2 -> Terminator110/1
  UDP Receive110/1 -> Display110/1
  UDP Receive111/2 -> Terminator111/1
  UDP Receive113/1 -> Display113/1
  UDP Receive112/2 -> Terminator112/1
  UDP Receive112/1 -> Display112/1
  UDP Receive113/2 -> Terminator113/1
  UDP Receive115/1 -> Display115/1
  UDP Receive114/2 -> Terminator114/1
  UDP Receive114/1 -> Display114/1
  UDP Receive115/2 -> Terminator115/1
  UDP Receive117/1 -> Display117/1
  UDP Receive116/2 -> Terminator116/1
  UDP Receive116/1 -> Display116/1
  UDP Receive117/2 -> Terminator117/1
  UDP Receive119/1 -> Display119/1
  UDP Receive118/2 -> Terminator118/1
  UDP Receive118/1 -> Display118/1
  UDP Receive119/2 -> Terminator119/1
